simulink model "formation_controller_pos3D_FIREanalysis_singleWPNAV"  (R2021a)
settings: Solver=VariableStepAuto  StartTime=0.0  StopTime=10.0  RelTol=1e-3
values from neighbouring files (symbols this model uses):
  collision_avoidance_activation_time = 2    [variables.m]
  delta1 = [0,5,10 ... (first row only)    [variables.m]
  delta2 = [-5,0,5 ... (first row only)    [variables.m]
  delta3 = [-10,-5,0 ... (first row only)    [variables.m]
  integral_init1 = [x0;y0;0]    [variables.m]
  integral_init2 = [x02;y02;0]    [variables.m]
  integral_init3 = [x03;y03;0]    [variables.m]
  kp_formation = 0.05    [variables.m]
  quota_volo_iniziale = -200    [variables.m]
  safety_region = 1    [variables.m]
  safety_region_control_gain = 0.1    [variables.m]
  safety_region_exp_scaler_beta = 2    [variables.m]
settings Model: Creator=fiori  LastModifiedBy=fiori
settings SolverCC: AlgebraicLoopSolver=TrustRegion
settings DebuggingCC: SFMachineParentedDataDiag=warning

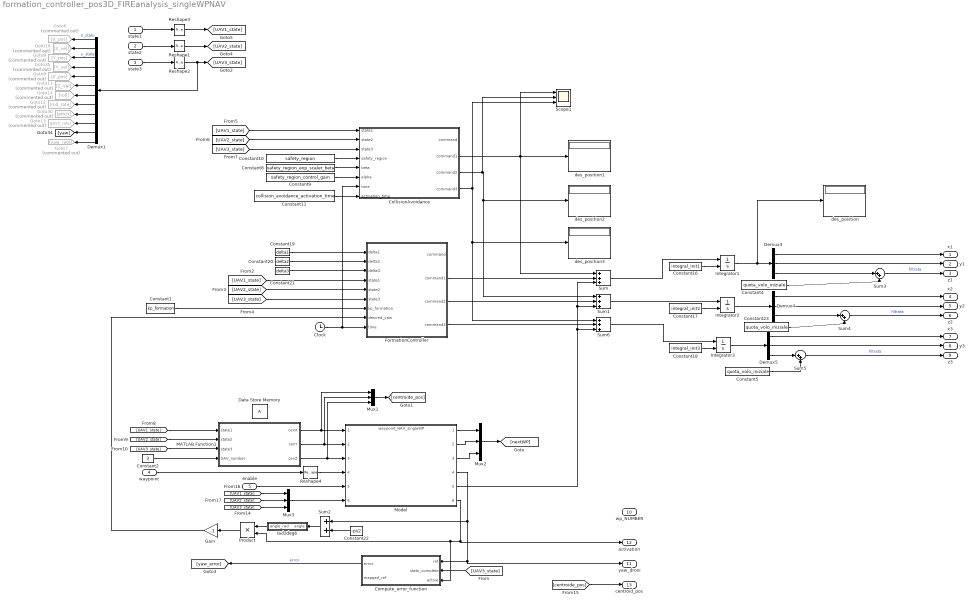
== system formation_controller_pos3D_FIREanalysis_singleWPNAV ==
  state1 : Inport
  state2 : Inport  Port=2
  state3 : Inport  Port=3
  waypoint : Inport  Port=4  PortDimensions=[3,1]
  enable : Inport  Port=5
  Clock : Clock
  CollisionAvoidance : MATLAB Function  TreatAsAtomicUnit=on
  Compute_error_function : MATLAB Function  TreatAsAtomicUnit=on
  Constant1 : Constant  Value=kp_formation
  Constant10 : Constant  Value=safety_region
  Constant11 : Constant  Value=collision_avoidance_activation_time
  Constant16 : Constant  Value=integral_init1
  Constant17 : Constant  Value=integral_init2
  Constant18 : Constant  Value=integral_init3
  Constant19 : Constant  Value=delta1
  Constant2 : Constant  Value=3
  Constant20 : Constant  Value=delta2
  Constant21 : Constant  Value=delta3
  Constant22 : Constant  Value=-pi/2
  Constant23 : Constant  Value=quota_volo_iniziale
  Constant4 : Constant  Value=quota_volo_iniziale
  Constant5 : Constant  Value=quota_volo_iniziale
  Constant8 : Constant  Value=safety_region_exp_scaler_beta
  Constant9 : Constant  Value=safety_region_control_gain
  Data Store Memory : DataStoreMemory  ReadBeforeWriteMsg=warning  WriteAfterWriteMsg=warning  WriteAfterReadMsg=warning  ShowAdditionalParam=off
  Demux1 : Demux  Outputs=12
  Demux3 : Demux  Outputs=3
  Demux4 : Demux  Outputs=3
  Demux5 : Demux  Outputs=3
  FormationController : MATLAB Function  TreatAsAtomicUnit=on
  Gain : Gain  Gain=-1
  Goto10 : Goto  Commented=on  GotoTag=X_vel
  Goto11 : Goto  Commented=on  GotoTag=Z_vel
  Goto12 : Goto  Commented=on  GotoTag=roll_rate
  Goto13 : Goto  Commented=on  GotoTag=pitch_rate
  Goto14 : Goto  Commented=on  GotoTag=roll
  Goto30 : Goto  Commented=on  GotoTag=pitch
  Goto35 : Goto  Commented=on  GotoTag=Y_vel
  Goto6 : Goto  Commented=on  GotoTag=X_pos
  Goto7 : Goto  Commented=on  GotoTag=yaw_rate
  Goto8 : Goto  Commented=on  GotoTag=Y_pos
  Goto9 : Goto  Commented=on  GotoTag=Z_pos
  Integrator1 : Integrator  InitialConditionSource=external  UpperSaturationLimit=3  LowerSaturationLimit=-3  IgnoreLimit=on
  Integrator2 : Integrator  InitialConditionSource=external  UpperSaturationLimit=3  LowerSaturationLimit=-3
  Integrator3 : Integrator  InitialConditionSource=external  UpperSaturationLimit=3  LowerSaturationLimit=-3
  MATLAB Function1 : MATLAB Function  TreatAsAtomicUnit=on
  Model : ModelReference  ModelNameDialog=waypoint_NAV_singleWP.slx  SimulationMode=Normal  ModelReferenceVersion=2.3
  Mux1 : Mux  Inputs=3
  Mux2 : Mux  Inputs=3
  Mux3 : Mux  Inputs=3
  Product : Product
  Reshape1 : Reshape  OutputDimensionality=Customize  OutputDimensions=[12,1]
  Reshape2 : Reshape  OutputDimensionality=Customize  OutputDimensions=[12,1]
  Reshape3 : Reshape  OutputDimensionality=Customize  OutputDimensions=[12,1]
  Reshape4 : Reshape  OutputDimensionality=Customize  OutputDimensions=[3,1]
  Scope1 : Scope  NumInputPorts=3
  Sum : Sum  Inputs=+|+|+
  Sum1 : Sum  Inputs=+|+|+
  Sum2 : Sum
  Sum3 : Sum  Inputs=|++
  Sum4 : Sum  Inputs=|++
  Sum5 : Sum  Inputs=|++
  Sum6 : Sum  Inputs=+|+|+
  des_position{,1..3} (4 alike) : Display
  rad2deg6 : MATLAB Function  TreatAsAtomicUnit=on
  x1 : Outport
  y1 : Outport  Port=2
  z1 : Outport  Port=3
  x2 : Outport  Port=4
  y2 : Outport  Port=5
  z2 : Outport  Port=6
  x3 : Outport  Port=7
  y3 : Outport  Port=8
  z3 : Outport  Port=9
  wp_NUMBER : Outport  Port=10
  yaw_droni : Outport  Port=11
  activation : Outport  Port=12
  centroid_pos : Outport  Port=13
  wires:
  Sum6/1 -> Integrator3/1
  MATLAB Function1/2(cenY) -> Mux1/2, Model/2
  Clock/1 -> CollisionAvoidance/7(time), FormationController/9(time)
  MATLAB Function1/3(cenZ) -> Mux1/3, Model/3
  Integrator2/1 -> Demux4/1
  Sum1/1 -> Integrator2/1
  Constant19/1 -> FormationController/1(delta1)
  MATLAB Function1/1(cenX) -> Mux1/1, Model/1
  Constant1/1 -> FormationController/7(kp_formation)
  Constant21/1 -> FormationController/3(delta3)
  Constant2/1 -> MATLAB Function1/4(UAV_number)
  state2/1 -> Reshape1/1
  state1/1 -> Reshape3/1
  Constant16/1 -> Integrator1/2
  state3/1 -> Reshape2/1
  Constant20/1 -> FormationController/2(delta2)
  Integrator3/1 -> Demux5/1
  FormationController/3(command2) -> Sum1/2
  Constant18/1 -> Integrator3/2
  Constant17/1 -> Integrator2/2
  Integrator1/1 -> des_position/1, Demux3/1
  Sum/1 -> Integrator1/1
  Demux3/1 -> x1/1
  Demux3/2 -> y1/1
  Demux4/1 -> x2/1
  Demux4/2 -> y2/1
  Demux5/2 -> y3/1
  Demux5/1 -> x3/1
  Demux3/3 -> Sum3/1
  Demux4/3 -> Sum4/1
  Demux5/3 -> Sum5/1
  Model/2 -> Mux2/2
  Model/1 -> Mux2/1
  Model/3 -> Mux2/3
  Mux2/1 -> [nextWP]
  Mux1/1 -> [centroide_pos]
  [UAV3_state] -> Compute_error_function/2(stato_completo)
  Compute_error_function/1(error) -> [yaw_error]  "error"
  Constant8/1 -> CollisionAvoidance/5(beta)
  Constant9/1 -> CollisionAvoidance/6(alpha)
  Reshape1/1 -> [UAV2_state]
  Reshape3/1 -> [UAV1_state]
  [UAV1_state] -> FormationController/4(state1)
  [UAV2_state] -> FormationController/5(state2)
  [UAV3_state] -> FormationController/6(state3)
  [UAV2_state] -> CollisionAvoidance/2(state2)
  [UAV1_state] -> CollisionAvoidance/1(state1)
  [UAV3_state] -> CollisionAvoidance/3(state3)
  Constant10/1 -> CollisionAvoidance/4(safety_region)
  FormationController/2(command1) -> Sum/2
  FormationController/4(command3) -> Sum6/2
  [UAV3_state] -> MATLAB Function1/3(state3)
  [UAV2_state] -> MATLAB Function1/2(state2)
  [UAV1_state] -> MATLAB Function1/1(state1)
  CollisionAvoidance/4(command3) -> des_position3/1, Sum6/1, Scope1/3
  CollisionAvoidance/3(command2) -> Scope1/2, des_position2/1, Sum1/1
  CollisionAvoidance/2(command1) -> Scope1/1, des_position1/1, Sum/1
  Constant11/1 -> CollisionAvoidance/8(activation_time)
  Sum2/1 -> rad2deg6/1(angle)
  Demux1/11 -> [yaw]
  Demux1/10 -> Goto13/1
  Demux1/9 -> Goto30/1
  Demux1/12 -> Goto7/1
  Demux1/8 -> Goto12/1
  Demux1/4 -> Goto35/1
  Demux1/1 -> Goto6/1  "X_stato"
  Demux1/7 -> Goto14/1
  Demux1/3 -> Goto8/1  "y_state"
  Demux1/2 -> Goto10/1
  Reshape2/1 -> Demux1/1, [UAV3_state]
  Demux1/5 -> Goto9/1
  Demux1/6 -> Goto11/1
  Model/4 -> Compute_error_function/1(ref), yaw_droni/1, Sum2/1
  Product/1 -> Gain/1
  rad2deg6/1(angle_rad) -> Product/1
  Constant22/1 -> Sum2/2
  Gain/1 -> FormationController/8(desired_yaw)
  waypoint/1 -> Reshape4/1
  Constant5/1 -> Sum5/2
  Constant23/1 -> Sum4/2
  Constant4/1 -> Sum3/2
  Model/6 -> Compute_error_function/3(active), Product/2, activation/1
  [centroide_pos] -> centroid_pos/1
  Sum3/1 -> z1/1  "filtrata"
  Sum4/1 -> z2/1  "filtrata"
  Sum5/1 -> z3/1  "filtrata"
  enable/1 -> Model/5
  Mux3/1 -> Model/6
  [UAV3_state] -> Mux3/3
  [UAV2_state] -> Mux3/2
  [UAV1_state] -> Mux3/1
  Model/5 -> Sum1/3, Sum/3, Sum6/3
  Reshape4/1 -> Model/4

== matlab function formation_controller_pos3D_FIREanalysis_singleWPNAV/MATLAB Function1 ==
  data: state1 input; cenX output; state2 input; state3 input; cenY output; cenZ output; UAV_number input
function [cenX,cenY,cenZ] = compute_centroide_position(state1,state2,state3,UAV_number)
    UAV1_state=[state1(1);state1(3);state1(5)];
    UAV2_state=[state2(1);state2(3);state2(5)];
    UAV3_state=[state3(1);state3(3);state3(5)];
    
    posizioni=[UAV1_state,UAV2_state,UAV3_state];
    sum_posizioni=[0;0;0];
    for i=1:3
        sum_posizioni = sum_posizioni + posizioni(:,i);
    end
    vettore=(1/UAV_number)*sum_posizioni;
    cenX=vettore(1);
    cenY=vettore(2);
    cenZ=vettore(3);
end

== matlab function formation_controller_pos3D_FIREanalysis_singleWPNAV/FormationController ==
  data: delta1 input; delta2 input; delta3 input; state1 input; command output; state2 input; state3 input; kp_formation input; desired_yaw input; time input; command1 output; command2 output; command3 output
function [command,command1,command2,command3] = formation_controller(delta1,delta2,delta3,state1,state2,state3,kp_formation,desired_yaw,time)
UAV1_state=[state1(1);state1(3);state1(5)];
UAV2_state=[state2(1);state2(3);state2(5)];
UAV3_state=[state3(1);state3(3);state3(5)];


posizioni=[UAV1_state,UAV2_state,UAV3_state];


somma=[0;0;0];
command=zeros(3,3);

psi=desired_yaw;
RZ= [cos(psi) sin(psi) 0; -sin(psi) cos(psi) 0; 0 0 1];

if time>=0
    for i=1:3
        if i==1
            for j=1:3
                somma=somma+posizioni(:,j)-posizioni(:,i)-(RZ*delta1(:,j));
            end
        elseif i==2
            for j=1:3
                somma=somma+posizioni(:,j)-posizioni(:,i)-(RZ*delta2(:,j));
            end
        else
            for j=1:3
                somma=somma+posizioni(:,j)-posizioni(:,i)-(RZ*delta3(:,j));
            end
        end
        
        if abs(somma(1))<0.1
            somma(1)=0;
        end
        if abs(somma(2))<0.1
            somma(2)=0;
        end
        if abs(somma(3))<0.1
            somma(3)=0;
        end
        command(:,i)=kp_formation*somma;
        somma=[0;0;0];
    end
end
command1=command(:,1);
command2=command(:,2);
command3=command(:,3);
end

== matlab function formation_controller_pos3D_FIREanalysis_singleWPNAV/CollisionAvoidance ==
  data: state1 input; state2 input; state3 input; safety_region input; command output; command1 output; command2 output; command3 output; beta input; alpha input; time input; activation_time input
function [command,command1,command2,command3] = formation_controller_COLLISION(state1,state2,state3,safety_region,beta,alpha,time,activation_time)
UAV1_state=[state1(1);state1(3);state1(5)];
UAV2_state=[state2(1);state2(3);state2(5)];
UAV3_state=[state3(1);state3(3);state3(5)];


posizioni=[UAV1_state,UAV2_state,UAV3_state];

somma=0;
command=zeros(1,3);


if time > activation_time
    for i=1:3
        for j=1:3
            if j==i
                valore=0;
            else 
                r_ij = posizioni(:,j) - posizioni(:,i);
                norma=norm(r_ij);
                if norma <= safety_region
                    valore = alpha * (exp(-beta*norma) - exp(-beta*safety_region));
                else
                    valore=0;
                end
            end
            somma=somma+valore;
        end
        command(:,i)=somma;
        somma=0;
    end

end
command1=command(:,1);
command2=command(:,2);
command3=command(:,3);
end

== matlab function formation_controller_pos3D_FIREanalysis_singleWPNAV/Compute_error_function ==
  data: ref input; error output; stato_completo input; mapped_ref output; active input
function [error,mapped_ref] = comp_error(ref,stato_completo,active)

state=stato_completo(11);

if active
    ref = ref - 2*pi*floor(ref/(2*pi));
    mapped_ref = ref;
        err = mapped_ref - state;

        if err > 0
            if err > pi
                err = err - 2*pi;
            end
        end

        if err < 0
            if err < -pi
                err = err + 2*pi;
            end
        end
        error=-err;
else 
    error=0;
    mapped_ref=0;
end

end

== matlab function formation_controller_pos3D_FIREanalysis_singleWPNAV/rad2deg6 ==
  data: angle input; angle_rad output
function angle_rad = fcn(angle)
    angle_rad = angle - 2*pi*floor(angle/(2*pi));
end
